simulink model "fourier_npu_algorithm"  (R2026a)
settings: Solver=FixedStepDiscrete  StopTime=0  FixedStep=1
undefined symbols (not defined in the file or in its folder): V4_INPUT

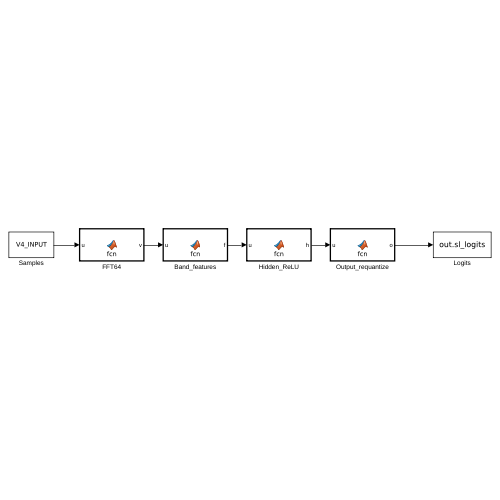
[thumbnail: Simulink's stored preview of the top-level diagram]
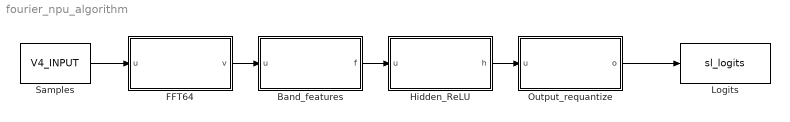
== system fourier_npu_algorithm ==
  Band_features : MATLAB Function  TreatAsAtomicUnit=on
  FFT64 : MATLAB Function  TreatAsAtomicUnit=on
  Hidden_ReLU : MATLAB Function  TreatAsAtomicUnit=on
  Logits : ToWorkspace  VariableName=sl_logits  SampleTime=-1
  Output_requantize : MATLAB Function  TreatAsAtomicUnit=on
  Samples : Constant  Value=V4_INPUT
  wires:
  Samples/1 -> FFT64/1(u)
  FFT64/1(v) -> Band_features/1(u)
  Band_features/1(f) -> Hidden_ReLU/1(u)
  Hidden_ReLU/1(h) -> Output_requantize/1(u)
  Output_requantize/1(o) -> Logits/1

== matlab function fourier_npu_algorithm/FFT64 ==
  data: u input; v output
function v=fcn(u)
v=fourier_fft_sl(u);
end

== matlab function fourier_npu_algorithm/Hidden_ReLU ==
  data: u input; h output
function h=fcn(u)
w=[20 -50 -20 2;18 -49 -20 11;-4 -3 12 -10;-34 79 21 -41];
b=[1490;1298;-427;1915];
h=max(0,min(127,floor((w*double(u(:))+b)/2^5)));
end

== matlab function fourier_npu_algorithm/Output_requantize ==
  data: u input; o output
function o=fcn(u)
w=[62 57 8 -65;-69 -67 5 56];
b=[-698;698];
o=max(-128,min(127,floor((w*double(u(:))+b)/2^6)));
end

== matlab function fourier_npu_algorithm/Band_features ==
  data: u input; f output
function f=fcn(u)
f=fourier_features_sl(u);
end
